simulink model "PD_elastic"  (R2021b)
settings: Solver=VariableStepAuto  StartTime=0.0  StopTime=30  RelTol=1e-3
undefined symbols (not defined in the file): Kd, Kp, qd
settings Model: Creator=fabioscap  LastModifiedBy=fabioscap

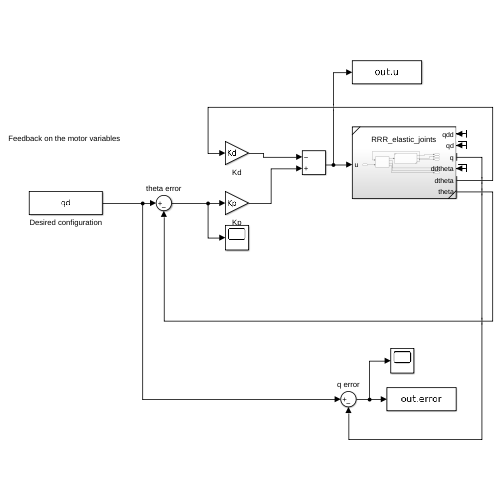
[thumbnail: Simulink's stored preview of the top-level diagram]
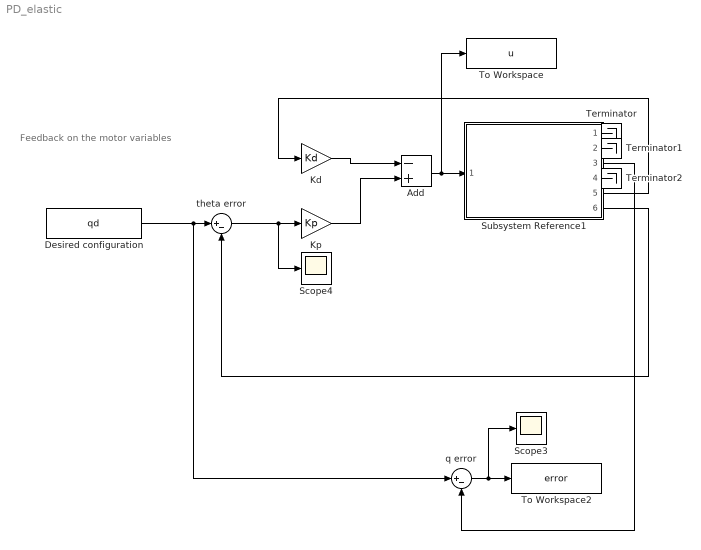
== system PD_elastic ==
  note: Feedback on the motor variables
  Add : Sum  Inputs=-+
  Desired configuration : Constant  Value=qd
  Kd : Gain  Gain=Kd
  Kp : Gain  Gain=Kp
  Scope3 : Scope
  Scope4 : Scope
  Subsystem Reference1 : Subsystem  ReferencedSubsystem=RRR_elastic_joints
  Terminator : Terminator
  Terminator1 : Terminator
  Terminator2 : Terminator
  To Workspace : ToWorkspace  VariableName=u  SaveFormat=Timeseries  SampleTime=-1
  To Workspace2 : ToWorkspace  VariableName=error  SaveFormat=Timeseries  SampleTime=-1
  q error : Sum  Inputs=|+-
  theta error : Sum  Inputs=|+-
  wires:
  Desired configuration/1 -> q error/1, theta error/1
  Kp/1 -> Add/2
  Kd/1 -> Add/1
  theta error/1 -> Scope4/1, Kp/1
  Subsystem Reference1/3 -> q error/2
  Subsystem Reference1/6 -> theta error/2
  Add/1 -> To Workspace/1, Subsystem Reference1/1
  Subsystem Reference1/5 -> Kd/1
  q error/1 -> Scope3/1, To Workspace2/1
  Subsystem Reference1/1 -> Terminator/1
  Subsystem Reference1/2 -> Terminator1/1
  Subsystem Reference1/4 -> Terminator2/1
